simulink model "DemoModel"  (R2020b)
settings: Solver=VariableStepAuto  StartTime=0.0  StopTime=10.0  RelTol=1e-3
PreLoadFcn:
  | ModelData;
undefined symbols (not defined in the file): Ki, Kp
settings Model: Creator=lehuahu  LastModifiedBy=lehuahu

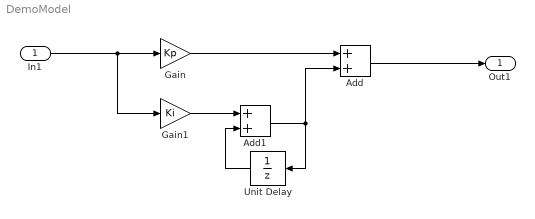
== system DemoModel ==
  In1 : Inport
  Add : Sum
  Add1 : Sum
  Gain : Gain  Gain=Kp
  Gain1 : Gain  Gain=Ki
  Unit Delay : UnitDelay  SampleTime=-1  HasFrameUpgradeWarning=on
  Out1 : Outport
  wires:
  In1/1 -> Gain1/1, Gain/1
  Gain/1 -> Add/1
  Add/1 -> Out1/1
  Gain1/1 -> Add1/1
  Unit Delay/1 -> Add1/2
  Add1/1 -> Unit Delay/1, Add/2
